simulink model "Lab2"  (R2014a)
settings: Solver=ode45  StartTime=0.0  StopTime=10.0  RelTol=1e-3
settings Model: Creator=Msi  LastModifiedBy=Msi

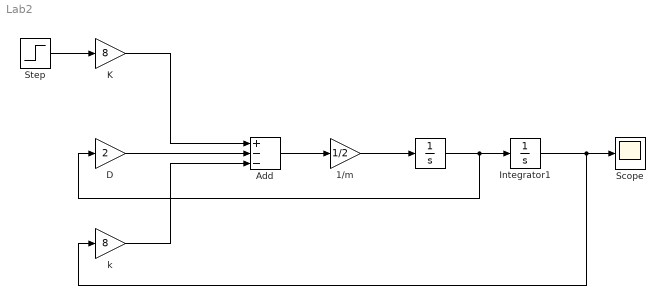
== system Lab2 ==
  " " : Integrator
  1/m : Gain  Gain=1/2
  Add : Sum  Inputs=+--
  D : Gain  Gain=2
  Integrator1 : Integrator
  K : Gain  Gain=8
  Scope : Scope
  Step : Step  SampleTime=0
  k : Gain  Gain=8
  wires:
  K/1 -> Add/1
  Step/1 -> K/1
  D/1 -> Add/2
  k/1 -> Add/3
  Add/1 -> 1/m/1
  1/m/1 -> " "/1
  " "/1 -> D/1, Integrator1/1
  Integrator1/1 -> k/1, Scope/1
